simulink model "FNM_05_Descentralizado_IMC"  (Simulink 7.1)
settings: Solver=ode45  StartTime=0.0  StopTime=3100  RelTol=1e-3
undefined symbols (not defined in the file or in its folder): analoginput, analogoutput, QT
libraries: daqlib x2
settings Model: Creator=didaticontrol  LastModifiedBy=didaticontrol

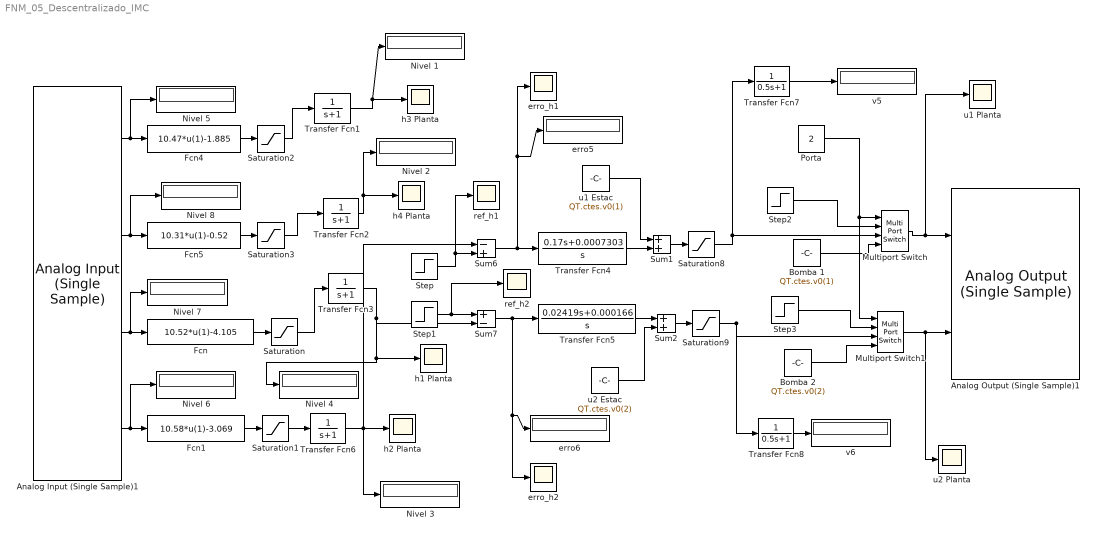
== system FNM_05_Descentralizado_IMC ==
  Analog Input (Single Sample)1 : daqlib/Analog Input (Single Sample)  DialogController=daqcreatedialog  DialogControllerArgs=DataTag0  DeviceMenu=nidaq Dev1 (USB-6008)  Device=nidaq Dev1 (USB-6008)  ObjConstructor=analoginput('nidaq','Dev1')  InputType=Differential  NChannelsSelected=4  Channels=1$0$$5$#1$1$$5$#1$2$$5$#1$3$$5$#  NPorts=1 per hardware channel  BlockSampleTime=10e-3
  Analog Output (Single Sample)1 : daqlib/Analog Output (Single Sample)  DialogController=daqcreatedialog  DialogControllerArgs=DataTag1  DeviceMenu=nidaq Dev1 (USB-6008)  Device=nidaq Dev1 (USB-6008)  ObjConstructor=analogoutput('nidaq','Dev1')  NChannelsSelected=2  Channels=1$0$$1$0$#1$1$$1$0$#  NPorts=1 per hardware channel
  Bomba 1 : Constant  Value=QT.ctes.v0(1)
  Bomba 2 : Constant  Value=QT.ctes.v0(2)
  Fcn : Fcn  Expr=10.52*u(1)-4.105  SampleTime=10e-3
  Fcn1 : Fcn  Expr=10.58*u(1)-3.069
  Fcn4 : Fcn  Expr=10.47*u(1)-1.885
  Fcn5 : Fcn  Expr=10.31*u(1)-0.52
  Multiport Switch : MultiPortSwitch  OutDataType=sfix(16)  OutScaling=2^0
  Multiport Switch1 : MultiPortSwitch  OutDataType=sfix(16)  OutScaling=2^0
  Nivel {1..8} (8 alike) : Display
  Porta : Constant  Value=2
  Saturation : Saturate  UpperLimit=23  LowerLimit=0  SampleTime=10e-3
  Saturation1 : Saturate  UpperLimit=23  LowerLimit=0
  Saturation2 : Saturate  UpperLimit=23  LowerLimit=0
  Saturation3 : Saturate  UpperLimit=23  LowerLimit=0
  Saturation8 : Saturate  UpperLimit=0.7*5  LowerLimit=0  SampleTime=10e-3
  Saturation9 : Saturate  UpperLimit=0.7*5  LowerLimit=0  SampleTime=10e-3
  Step : Step  Time=2300  Before=QT.ctes.h0(2)  After=QT.ctes.h0(2)+1
  Step1 : Step  Time=1500  Before=QT.ctes.h0(1)  After=QT.ctes.h0(1)+1
  Step2 : Step  Time=50  Before=QT.ctes.v0(1)  After=QT.ctes.v0(1)  SampleTime=10e-3
  Step3 : Step  Time=50  Before=QT.ctes.v0(2)  After=QT.ctes.v0(2)
  Sum1 : Sum  OutDataType=sfix(16)  OutScaling=2^0
  Sum2 : Sum  OutDataType=sfix(16)  OutScaling=2^0
  Sum6 : Sum  Inputs=-+  OutDataType=sfix(16)  OutScaling=2^0
  Sum7 : Sum  Inputs=+-  OutDataType=sfix(16)  OutScaling=2^0
  Transfer Fcn{1..3,6} (4 alike) : TransferFcn  Denominator=[1 1]
  Transfer Fcn4 : TransferFcn  Numerator=[0.17 0.0007303]  Denominator=[1 0]
  Transfer Fcn5 : TransferFcn  Numerator=[0.02419 0.000166]  Denominator=[1 0]
  Transfer Fcn7 : TransferFcn  Denominator=[0.5 1]
  Transfer Fcn8 : TransferFcn  Denominator=[0.5 1]
  erro5 : Display
  erro6 : Display
  erro_h1 : Scope
      settings: TimeRange=300  YMin=0  YMax=9.5  SaveName=erro_h1  SampleInput=on  SampleTime=10e-3
  erro_h2 : Scope
      settings: TimeRange=300  YMin=0  YMax=9.5  SaveName=erro_h2  SampleInput=on  SampleTime=10e-3
  h1 Planta : Scope
      settings: YMin=0  YMax=10  SaveName=h1_real  SampleInput=on  SampleTime=10e-3
  h2 Planta : Scope
      settings: YMin=0  YMax=10.5  SaveName=h2_real  SampleInput=on  SampleTime=10e-3
  h3 Planta : Scope
      settings: YMin=0  YMax=10.5  SaveName=h3_real  SampleInput=on  SampleTime=10e-3
  h4 Planta : Scope
      settings: YMin=0  YMax=10.5  SaveName=h4_real  SampleInput=on  SampleTime=10e-3
  ref_h1 : Scope
      settings: TimeRange=300  YMin=0  YMax=9.5  SaveName=ref_h1  SampleInput=on  SampleTime=10e-3
  ref_h2 : Scope
      settings: TimeRange=300  YMin=0  YMax=9.5  SaveName=ref_h2  SampleInput=on  SampleTime=10e-3
  u1 Planta : Scope
      settings: YMin=1.2  YMax=3.5  SaveName=u1_real  SampleInput=on  SampleTime=10e-3
  u1 Estac : Constant  Value=QT.ctes.v0(1)
  u2 Planta : Scope
      settings: YMin=1.7  YMax=3.5  SaveName=u2_real  SampleInput=on  SampleTime=10e-3
  u2 Estac : Constant  Value=QT.ctes.v0(2)
  v5 : Display
  v6 : Display
  wires:
  Analog Input (Single Sample)1/3 -> Fcn/1, Nivel 7/1
  Fcn/1 -> Saturation/1
  Fcn1/1 -> Saturation1/1
  Analog Input (Single Sample)1/4 -> Fcn1/1, Nivel 6/1
  Analog Input (Single Sample)1/2 -> Fcn5/1, Nivel 8/1
  Analog Input (Single Sample)1/1 -> Nivel 5/1, Fcn4/1
  Fcn4/1 -> Saturation2/1
  Fcn5/1 -> Saturation3/1
  Multiport Switch1/1 -> Analog Output (Single Sample)1/2, u2 Planta/1
  Sum6/1 -> erro5/1, erro_h1/1, Transfer Fcn4/1
  Sum7/1 -> erro6/1, erro_h2/1, Transfer Fcn5/1
  Saturation9/1 -> Transfer Fcn8/1, Multiport Switch1/3
  Step/1 -> Sum6/2, ref_h1/1
  Step1/1 -> Sum7/1, ref_h2/1
  Sum1/1 -> Saturation8/1
  Transfer Fcn4/1 -> Sum1/2
  u1 Estac/1 -> Sum1/1
  Sum2/1 -> Saturation9/1
  u2 Estac/1 -> Sum2/2
  Multiport Switch/1 -> u1 Planta/1, Analog Output (Single Sample)1/1
  Saturation8/1 -> Transfer Fcn7/1, Multiport Switch/3
  Transfer Fcn1/1 -> h3 Planta/1, Nivel 1/1
  Saturation2/1 -> Transfer Fcn1/1
  Transfer Fcn2/1 -> Nivel 2/1, h4 Planta/1
  Saturation3/1 -> Transfer Fcn2/1
  Transfer Fcn3/1 -> Nivel 4/1, h1 Planta/1, Sum7/2
  Saturation/1 -> Transfer Fcn3/1
  Transfer Fcn6/1 -> h2 Planta/1, Nivel 3/1, Sum6/1
  Saturation1/1 -> Transfer Fcn6/1
  Transfer Fcn7/1 -> v5/1
  Transfer Fcn8/1 -> v6/1
  Porta/1 -> Multiport Switch/1, Multiport Switch1/1
  Bomba 1/1 -> Multiport Switch/4
  Bomba 2/1 -> Multiport Switch1/4
  Step3/1 -> Multiport Switch1/2
  Step2/1 -> Multiport Switch/2
  Transfer Fcn5/1 -> Sum2/1
